simulink model "howard_lin_r2013a_20160129"  (R2013a)
settings: Solver=ode45  StartTime=0.0  StopTime=tFinal  RelTol=1e-3
PreLoadFcn:
  | OAT=30;
  | Temp=68;
  | 
  | Rn=29;
  | Rx=69;
  | Tn=180;
  | Tx=120;
  | 
  | Hc=114/86400;
  | Ha=1.61/86400;
  | %Hf=1.08/86400;
  | Hf=1.745/86400;
  | Ho=283/86400;
  | 
  | tau=40;
  | FILTER_DELAY = 5;
  | 
  | Kv=400;  % gain in TCOMP of house control
  | Kei=2e-4;
  | Kep=1;
  | 
  | % From match to thermo20160128.xlsx
  | sNoise=0.001;
  | SET = [0 60 18861 18862; 68 62 68 68]';
  | otherHeat=[0 1000 6000; .001 .001 .0005]';
  | tFinal = 24132;
InitFcn:
  | Ta0=Temp;
  | Tw0 = (Temp*Ha + OAT*Ho)/(Ho+Ha);
  | Tb0=max(min(interp1([Rn Rx],[Tn Tx],OAT), Tn),Tx);
  | Tc0 = ((Ha+Hc)*Ta0 - Ha*Tw0) / Hc;
  | D0 =max(min( Hc*(Tc0-Ta0)/(Hf*(Tb0-Tc0)), 1), 1e-32);
  | intEi = 0.2;
  | intEo=0;
settings Model: Creator=210023782  LastModifiedBy=210023782
settings DataIOCC: InitialState=xinHouse  LimitDataPoints=off  SaveState=on  StateSaveName=xoutHouse

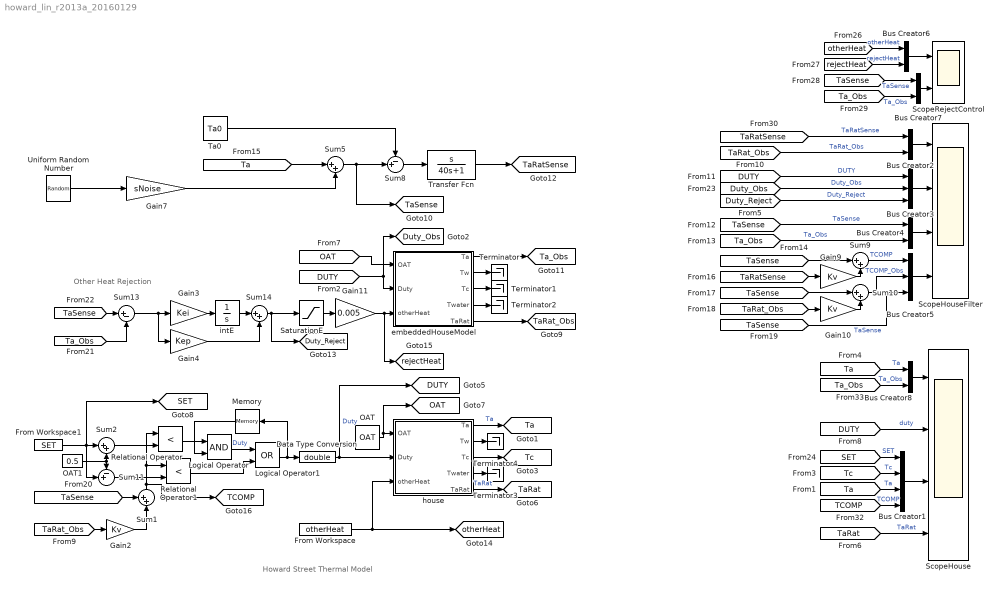
== system howard_lin_r2013a_20160129 ==
  note: Howard Street Thermal Model
  note: Other Heat Rejection
  Bus Creator1 : BusCreator
  Bus Creator{2,4,6..8} (5 alike) : BusCreator  Inputs=2
  Bus Creator3 : BusCreator  Inputs=3
  Bus Creator5 : BusCreator  Inputs=3
  Data Type Conversion : DataTypeConversion  OutDataTypeStr=double
  From Workspace : FromWorkspace  VariableName=otherHeat  SampleTime=1  OutputAfterFinalValue=Holding final value
  From Workspace1 : FromWorkspace  VariableName=SET  SampleTime=1  OutputAfterFinalValue=Holding final value
  Gain10 : Gain  Gain=Kv
  Gain11 : Gain  Gain=0.005
  Gain2 : Gain  Gain=Kv
  Gain3 : Gain  Gain=Kei
  Gain4 : Gain  Gain=Kep
  Gain7 : Gain  Gain=sNoise
  Gain9 : Gain  Gain=Kv
  Logical Operator : Logic  AllPortsSameDT=off  OutDataTypeStr=boolean
  Logical Operator1 : Logic  Operator=OR  AllPortsSameDT=off  OutDataTypeStr=boolean
  Memory : Memory
  OAT : Constant  Value=OAT
  OAT1 : Constant  Value=0.5
  Relational Operator : RelationalOperator  Operator=<  OutDataTypeStr=boolean
  Relational Operator1 : RelationalOperator  Operator=<  OutDataTypeStr=boolean
  SaturationE : Saturate  UpperLimit=1  LowerLimit=-1
  ScopeHouse : Scope  NumInputPorts=4
      settings: ShowLegends=on  YMin=-75~-40~-5~-5  YMax=75~70~5~5  Decimation=2
  ScopeHouseFilter : Scope  NumInputPorts=4
      settings: ShowLegends=on  YMin=-75~-40~-10~-5  YMax=75~70~10~5  SaveName=ScopeData4  Decimation=2
  ScopeRejectControl : Scope  NumInputPorts=2
      settings: ShowLegends=on  YMin=-75~-40  YMax=75~70  Decimation=2
  Sum1 : Sum  Inputs=++|
  Sum{2,5,9..10,14} (5 alike) : Sum  Inputs=|++
  Sum11 : Sum  Inputs=-+|
  Sum13 : Sum  Inputs=|+-
  Sum8 : Sum  Inputs=-+|
  Ta0 : Constant  Value=Ta0
  Terminator{,1..4} (5 alike) : Terminator
  Transfer Fcn : TransferFcn  Numerator=[1 0]  Denominator=[40 1]
  Uniform Random Number : UniformRandomNumber  SampleTime=FILTER_DELAY
  embeddedHouseModel : Subsystem
  house : Subsystem
  intE : Integrator  InitialCondition=intEi  LimitOutput=on  UpperSaturationLimit=1  LowerSaturationLimit=-1
  tag scope: DUTY=global, Duty_Obs=global, Duty_Reject=global, OAT=global, SET=global, TCOMP=global, Ta=global, TaRat=global, TaRatSense=global, TaRat_Obs=global, TaSense=global, Ta_Obs=global, Tc=global, otherHeat=global, rejectHeat=global
  wires:
  OAT/1 -> [OAT], house/1(OAT)
  house/1(Ta) -> [Ta]  "Ta"
  house/2(Tw) -> Terminator4/1
  house/3(Tc) -> [Tc]
  house/4(Twater) -> Terminator3/1
  Bus Creator2/1 -> ScopeHouseFilter/1
  house/5(TaRat) -> [TaRat]  "TaRat"
  [TaRat] -> ScopeHouse/4  "TaRat"
  Logical Operator/1 -> Logical Operator1/1  "Duty"
  Gain2/1 -> Sum1/2
  [OAT] -> embeddedHouseModel/1(OAT)
  [DUTY] -> [Duty_Obs], embeddedHouseModel/2(Duty)
  [TaRat_Obs] -> Gain2/1
  embeddedHouseModel/5(TaRat) -> [TaRat_Obs]
  embeddedHouseModel/2(Tw) -> Terminator/1
  embeddedHouseModel/3(Tc) -> Terminator1/1
  embeddedHouseModel/4(Twater) -> Terminator2/1
  Uniform Random Number/1 -> Gain7/1
  Sum5/1 -> [TaSense], Sum8/2
  Transfer Fcn/1 -> [TaRatSense]
  [TaRat_Obs] -> Bus Creator2/2  "TaRat_Obs"
  [DUTY] -> Bus Creator3/1  "DUTY"
  Bus Creator3/1 -> ScopeHouseFilter/2
  [Ta] -> Sum5/1
  Gain7/1 -> Sum5/2
  Ta0/1 -> Sum8/1
  Sum8/1 -> Transfer Fcn/1
  [TaSense] -> Bus Creator4/1  "TaSense"
  [Ta_Obs] -> Bus Creator4/2  "Ta_Obs"
  Bus Creator4/1 -> ScopeHouseFilter/3
  Bus Creator5/1 -> ScopeHouseFilter/4
  [TaRatSense] -> Gain9/1
  [TaSense] -> Sum9/1
  Gain9/1 -> Sum9/2
  Sum9/1 -> Bus Creator5/1  "TCOMP"
  [TaRat_Obs] -> Gain10/1
  [TaSense] -> Sum10/1
  Gain10/1 -> Sum10/2
  Sum10/1 -> Bus Creator5/2  "TCOMP_Obs"
  [TaSense] -> Bus Creator5/3  "TaSense"
  Sum1/1 -> [TCOMP], Relational Operator1/1, Relational Operator/1
  OAT1/1 -> Sum2/2, Sum11/1
  Sum2/1 -> Relational Operator/2
  [TaSense] -> Sum1/1
  Data Type Conversion/1 -> house/2(Duty), [DUTY]  "Duty"
  Relational Operator1/1 -> Logical Operator1/2
  Sum11/1 -> Relational Operator1/2
  From Workspace/1 -> house/3(otherHeat), [otherHeat]
  embeddedHouseModel/1(Ta) -> [Ta_Obs]
  Sum13/1 -> Gain3/1, Gain4/1
  Gain3/1 -> intE/1
  [Duty_Obs] -> Bus Creator3/2  "Duty_Obs"
  Logical Operator1/1 -> Memory/1, Data Type Conversion/1
  [DUTY] -> ScopeHouse/2  "duty"
  From Workspace1/1 -> [SET], Sum11/2, Sum2/1
  [Ta] -> Bus Creator1/3  "Ta"
  [Tc] -> Bus Creator1/2  "Tc"
  [SET] -> Bus Creator1/1  "SET"
  Bus Creator1/1 -> ScopeHouse/3
  [TaSense] -> Sum13/1
  [Ta_Obs] -> Sum13/2
  Sum14/1 -> [Duty_Reject], SaturationE/1
  [Duty_Reject] -> Bus Creator3/3  "Duty_Reject"
  [otherHeat] -> Bus Creator6/1  "otherHeat"
  Bus Creator6/1 -> ScopeRejectControl/1
  [rejectHeat] -> Bus Creator6/2  "rejectHeat"
  [TaSense] -> Bus Creator7/1  "TaSense"
  [Ta_Obs] -> Bus Creator7/2  "Ta_Obs"
  Bus Creator7/1 -> ScopeRejectControl/2
  intE/1 -> Sum14/1
  Gain4/1 -> Sum14/2
  Gain11/1 -> [rejectHeat], embeddedHouseModel/3(otherHeat)
  SaturationE/1 -> Gain11/1
  [TCOMP] -> Bus Creator1/4  "TCOMP"
  [Ta] -> Bus Creator8/1  "Ta"
  [Ta_Obs] -> Bus Creator8/2  "Ta_Obs"
  Bus Creator8/1 -> ScopeHouse/1
  [TaRatSense] -> Bus Creator2/1  "TaRatSense"
  Relational Operator/1 -> Logical Operator/2
  Memory/1 -> Logical Operator/1

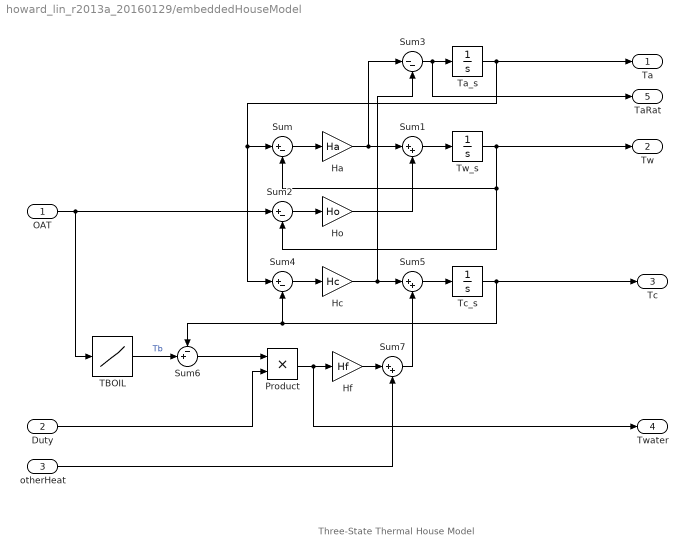
== system howard_lin_r2013a_20160129/embeddedHouseModel ==
  note: Three-State Thermal House Model
  OAT : Inport
  Duty : Inport  Port=2
  otherHeat : Inport  Port=3
  Ha : Gain  Gain=Ha
  Hc : Gain  Gain=Hc
  Hf : Gain  Gain=Hf
  Ho : Gain  Gain=Ho
  Product : Product
  Sum : Sum  Inputs=|+-
  Sum1 : Sum  Inputs=|++
  Sum2 : Sum  Inputs=|+-
  Sum3 : Sum  Inputs=|--
  Sum4 : Sum  Inputs=|+-
  Sum5 : Sum  Inputs=|++
  Sum6 : Sum  Inputs=-+|
  Sum7 : Sum  Inputs=|++
  TBOIL : Lookup_n-D  NumberOfTableDimensions=1  BreakpointsForDimension1=[Rn Rx]  Table=[Tn Tx]  ExtrapMethod=Clip  RndMeth=Simplest  InputSameDT=on
  Ta_s : Integrator  InitialCondition=Ta0
  Tc_s : Integrator  InitialCondition=Tc0
  Tw_s : Integrator  InitialCondition=Tw0
  Ta : Outport
  Tw : Outport  Port=2
  Tc : Outport  Port=3
  Twater : Outport  Port=4
  TaRat : Outport  Port=5
  wires:
  OAT/1 -> Sum2/1, TBOIL/1
  otherHeat/1 -> Sum7/2
  Sum7/1 -> Sum5/2
  Hf/1 -> Sum7/1
  TBOIL/1 -> Sum6/2  "Tb"
  Sum6/1 -> Product/1
  Duty/1 -> Product/2
  Product/1 -> Hf/1, Twater/1
  Hc/1 -> Sum5/1, Sum3/2
  Tc_s/1 -> Sum4/2, Sum6/1, Tc/1
  Sum5/1 -> Tc_s/1
  Sum3/1 -> Ta_s/1, TaRat/1
  Sum1/1 -> Tw_s/1
  Ho/1 -> Sum1/2
  Sum4/1 -> Hc/1
  Ha/1 -> Sum1/1, Sum3/1
  Tw_s/1 -> Sum2/2, Sum/2, Tw/1
  Sum2/1 -> Ho/1
  Sum/1 -> Ha/1
  Ta_s/1 -> Sum/1, Sum4/1, Ta/1

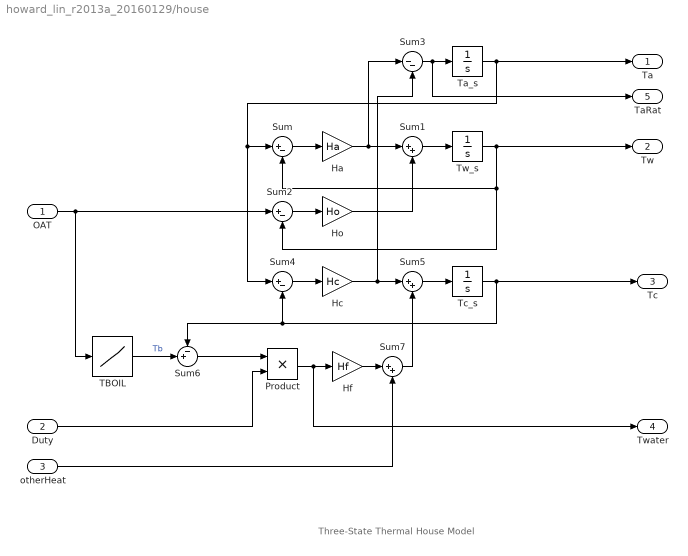
== system howard_lin_r2013a_20160129/house ==
  note: Three-State Thermal House Model
  OAT : Inport
  Duty : Inport  Port=2
  otherHeat : Inport  Port=3
  Ha : Gain  Gain=Ha
  Hc : Gain  Gain=Hc
  Hf : Gain  Gain=Hf
  Ho : Gain  Gain=Ho
  Product : Product
  Sum : Sum  Inputs=|+-
  Sum1 : Sum  Inputs=|++
  Sum2 : Sum  Inputs=|+-
  Sum3 : Sum  Inputs=|--
  Sum4 : Sum  Inputs=|+-
  Sum5 : Sum  Inputs=|++
  Sum6 : Sum  Inputs=-+|
  Sum7 : Sum  Inputs=|++
  TBOIL : Lookup_n-D  NumberOfTableDimensions=1  BreakpointsForDimension1=[Rn Rx]  Table=[Tn Tx]  ExtrapMethod=Clip  RndMeth=Simplest  InputSameDT=on
  Ta_s : Integrator  InitialCondition=Ta0
  Tc_s : Integrator  InitialCondition=Tc0
  Tw_s : Integrator  InitialCondition=Tw0
  Ta : Outport
  Tw : Outport  Port=2
  Tc : Outport  Port=3
  Twater : Outport  Port=4
  TaRat : Outport  Port=5
  wires:
  Ta_s/1 -> Ta/1, Sum4/1, Sum/1
  Sum/1 -> Ha/1
  Sum2/1 -> Ho/1
  Tw_s/1 -> Tw/1, Sum/2, Sum2/2
  Ha/1 -> Sum3/1, Sum1/1
  Sum4/1 -> Hc/1
  Ho/1 -> Sum1/2
  Sum1/1 -> Tw_s/1
  Sum3/1 -> TaRat/1, Ta_s/1
  Sum5/1 -> Tc_s/1
  Tc_s/1 -> Tc/1, Sum6/1, Sum4/2
  Hc/1 -> Sum3/2, Sum5/1
  Product/1 -> Twater/1, Hf/1
  Duty/1 -> Product/2
  Sum6/1 -> Product/1
  TBOIL/1 -> Sum6/2  "Tb"
  Hf/1 -> Sum7/1
  Sum7/1 -> Sum5/2
  otherHeat/1 -> Sum7/2
  OAT/1 -> TBOIL/1, Sum2/1
